simulink model "Safety_filter_obstacle_run"  (R2021b)
settings: Solver=ode4  StartTime=0.0  StopTime=30  FixedStep=0.01  RelTol=1e-3
settings Model: PacingRate=0.500000  Creator=14244039  LastModifiedBy=40335991
settings DebuggingCC: UnderSpecifiedDimensionMsg=warning

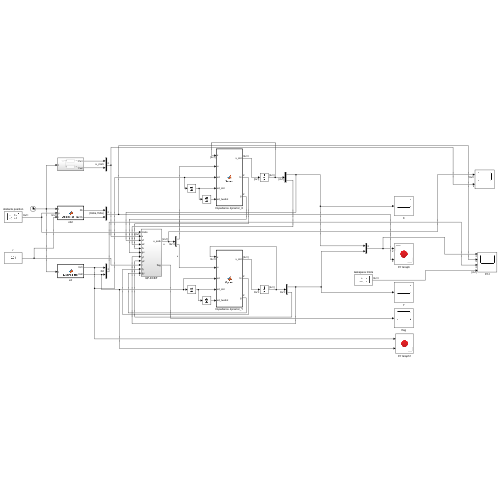
[thumbnail: Simulink's stored preview of the top-level diagram]
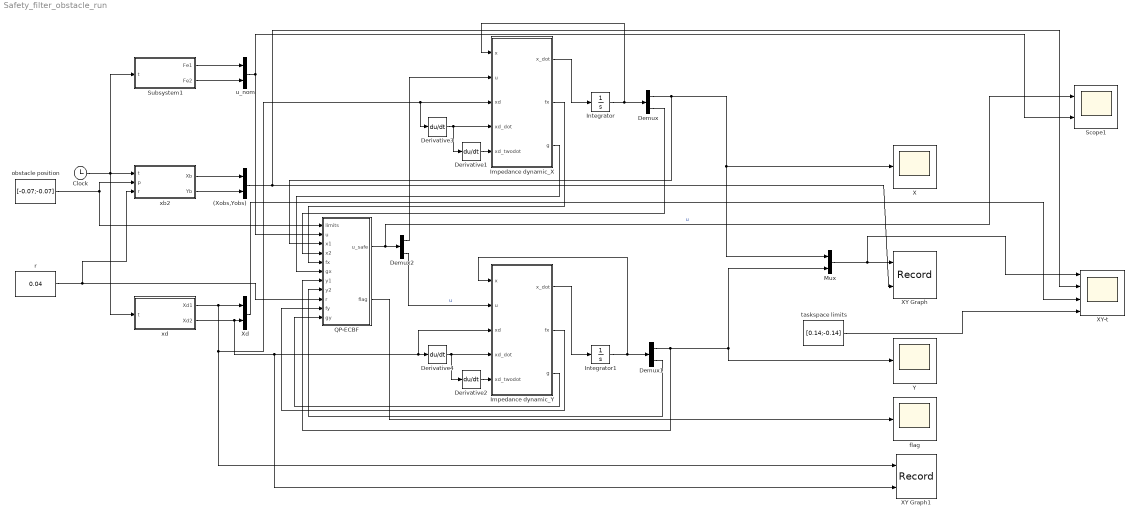
== system Safety_filter_obstacle_run ==
  (Xobs,Yobs) : Mux  Inputs=2
  Clock : Clock
  Demux : Demux  Outputs=2
  Demux1 : Demux  Outputs=2
  Demux2 : Demux  Outputs=2
  Derivative{1..4} (4 alike) : Derivative
  Impedance dynamic_X : MATLAB Function  TreatAsAtomicUnit=on
  Impedance dynamic_Y : MATLAB Function  TreatAsAtomicUnit=on
  Integrator : Integrator  InitialCondition=[0.14;0]
  Integrator1 : Integrator  InitialCondition=[0;0]
  Mux : Mux  Inputs=2
  QP-ECBF : Subsystem
  Scope1 : Scope  NumInputPorts=2
  Subsystem1 : Subsystem
  X : Scope
  XY Graph : Record  FileSettingsInternal="{\"entries\":[{\"content\":{\"excelSettings\":{\"content\":{},\"type\":\"Streamout.ExcelSettings\"}},\"type\":\"Streamout.FileSettingStorage\",\"uuid\":\"2cb9fd5d-0c84-4006-89a3-e297fa6ee1b5\"}],\"packageUris\":[\"http://schema.mathworks.com/mf0/streamout_blocks/R2020a\"],\"version\":\"1.0\"}"  Layout=[1 1]  SignalsInternal="{\"entries\":[{\"content\":{\"signals\":[{\"content\":{\"blockPath\":[\"Safety_filter_obstacle_run/XY Graph\"],\"channel\":[],\"dimensions\":[2],\"domain\":\"Safety_filter_obstacle_run/XY Graph\",\"hasChildren\":true,\"lineColor\":\"#fe330a\",\"plots\":[],\"port\":1,\"sid\":[\"\"],\"signalID\":5016,\"signalName\":\"Mux\"},\"type\":\"RecordBlkView.Signal\",\"uuid\":\"6b362bb2-f6dd-4a03-85b8-156c16026f8e\"},{\"content\":{\"blockPath\":[\"Safety_filter_obstacle_run/XY Graph\"],\"channel\":[1],\"dimensions\":[2],\"domain\":\"Safety_filter_obstacle_run/XY Graph\",\"lineColor\":\"#d95319\",\"parentID\":5016,\"plots\":[1],\"port\":1,\"sid\":[\"\"],\"signalID\":5017,\"signalName\":\"Mux\"},\"type\":\"RecordBlkView.Signal\",\"uuid\":\"500ae97e-7081-4371-a208-a6de7c56ece4\"},{\"content\":{\"blockPath\":[\"Safety_filter_obstacle_run/XY Graph\"],\"channel\":[],\"dimensions\":[2],\"domain\":\"Safety_filter_obstacle_run/XY Graph\",\"hasChildren\":true,\"lineColor\":\"#0072bd\",\"plots\":[],\"port\":2,\"sid\":[\"\"],\"signalID\":5021,\"signalName\":\"(Xobs,Yobs)\"},\"type\":\"RecordBlkView.Signal\",\"uuid\":\"f31b4382-cf55-47a1-8b18-86527234a350\"},{\"content\":{\"blockPath\":[\"Safety_filter_obstacle_run/XY Graph\"],\"channel\":[1],\"dimensions\":[2],\"domain\":\"Safety_filter_obstacle_run/XY Graph\",\"lineColor\":\"#7e2f8e\",\"parentID\":5021,\"plots\":[1],\"port\":2,\"sid\":[\"\"],\"signalID\":5022,\"signalName\":\"(Xobs,Yobs)\"},\"type\":\"RecordBlkView.Signal\",\"uuid\":\"742af8a8-3d57-45a7-b4dd-15d9969bab4c\"},{\"content\":{\"blockPath\":[\"Safety_filter_obstacle_run/XY Graph\"],\"channel\":[2],\"dimensions\":[2],\"domain\":\"Safety_filter_obstacle_run/XY Graph\",\"lineColor\":\"#a2142f\",\"parentID\":5016,\"plots\":[1],\"port\":1,\"sid\":[\"\"],\"signalID\":5035,\"signalName\":\"Mux\"},\"type\":\"RecordBlkView.Signal\",\"uuid\":\"5f11a2ec-fe27-4e67-93d5-fd7bb7e6a2c3\"},{\"content\":{\"blockPath\":[\"Safety_filter_obstacle_run/XY Graph\"],\"channel\":[2],\"dimensions\":[2],\"domain\":\"Safety_filter_obstacle_run/XY Graph\",\"lineColor\":\"#139fff\",\"parentID\":5021,\"plots\":[1],\"port\":2,\"sid\":[\"\"],\"signalID\":5036,\"signalName\":\"(Xobs,Yobs)\"},\"type\":\"RecordBlkView.Signal\",\"uuid\":\"66022486-a783-44e2-b1af-9294e060b914\"}]},\"type\":\"RecordBlkView.InputSignals\",\"uuid\":\"045e9bd8-92bd-4ba2-811b-fb3cc024f96b\"}],\"packageUris\":[\"http://schema.mathworks.com/mf0/streamout_blocks/R2020a\"],\"version\":\"1.0\"}"  VisualizationBindings="{\"xyplotplugin\":{\"info\":[{\"series\":[{\"bindingParametersList\":[{\"parameter\":\"X-Axis\",\"signalID\":5022,\"signalName\":\"(Xobs,Yobs)(1)\"},{\"parameter\":\"Y-Axis\",\"signalID\":5036,\"signalName\":\"(Xobs,Yobs)(2)\"}],\"seriesID\":588},{\"bindingParametersList\":[{\"parameter\":\"X-Axis\",\"signalID\":5017,\"signalName\":\"Mux(1)\"},{\"parameter\":\"Y-Axis\",\"signalID\":5035,\"signalName\":\"Mux(2)\"}],\"seriesID\":13609}],\"subplotID\":1}]}}"  CompatibilityTag=XY  st=-1
  XY Graph1 : Record  FileSettingsInternal="{\"entries\":[{\"content\":{\"excelSettings\":{\"content\":{},\"type\":\"Streamout.ExcelSettings\"}},\"type\":\"Streamout.FileSettingStorage\",\"uuid\":\"2cef4229-92dc-4655-bad0-2b3161d59ac8\"}],\"packageUris\":[\"http://schema.mathworks.com/mf0/streamout_blocks/R2020a\"],\"version\":\"1.0\"}"  Layout=[1 1]  SignalsInternal="{\"entries\":[{\"content\":{\"signals\":[{\"content\":{\"blockPath\":[\"Safety_filter_obstacle_run/XY Graph1\"],\"channel\":[],\"dimensions\":[1],\"domain\":\"Safety_filter_obstacle_run/XY Graph1\",\"lineColor\":\"#a2142f\",\"plots\":[1],\"port\":1,\"sid\":[\"\"],\"signalID\":5026,\"signalName\":\"xd:1\"},\"type\":\"RecordBlkView.Signal\",\"uuid\":\"d43ebe69-de7a-456f-bba9-24daebe6bc4b\"},{\"content\":{\"blockPath\":[\"Safety_filter_obstacle_run/XY Graph1\"],\"channel\":[],\"dimensions\":[1],\"domain\":\"Safety_filter_obstacle_run/XY Graph1\",\"lineColor\":\"#139fff\",\"plots\":[1],\"port\":2,\"sid\":[\"\"],\"signalID\":5030,\"signalName\":\"xd:2\"},\"type\":\"RecordBlkView.Signal\",\"uuid\":\"3ab767b2-3981-4008-8a03-ee9b94162d99\"}]},\"type\":\"RecordBlkView.InputSignals\",\"uuid\":\"ec3b1ac5-575a-40f9-bce4-3baa89b708d6\"}],\"packageUris\":[\"http://schema.mathworks.com/mf0/streamout_blocks/R2020a\"],\"version\":\"1.0\"}"  VisualizationBindings="{\"xyplotplugin\":{\"info\":[{\"series\":[{\"bindingParametersList\":[{\"parameter\":\"X-Axis\",\"signalID\":5026,\"signalName\":\"xd:1\"},{\"parameter\":\"Y-Axis\",\"signalID\":5030,\"signalName\":\"xd:2\"}],\"seriesID\":51409}],\"subplotID\":1}]}}"  CompatibilityTag=XY
  XY-t : Scope  NumInputPorts=4
  Xd : Mux  Inputs=2
  Y : Scope
  flag : Scope
  obstacle position : Constant  Value=[-0.07;-0.07]  VectorParams1D=off  SampleTime=-1
  r : Constant  Value=0.04  VectorParams1D=off  SampleTime=-1
  taskspace limits : Constant  Value=[0.14;-0.14]  VectorParams1D=off  SampleTime=-1
  u_nom : Mux  Inputs=2
  xb2 : MATLAB Function  TreatAsAtomicUnit=on
  xd : MATLAB Function  TreatAsAtomicUnit=on
  wires:
  Subsystem1/1(Fe1) -> u_nom/1
  Clock/1 -> xd/1(t), xb2/1(t), Subsystem1/1(t)
  Derivative3/1 -> Impedance dynamic_X/4(xd_dot), Derivative1/1
  Derivative1/1 -> Impedance dynamic_X/5(xd_twodot)
  Impedance dynamic_X/1(x_dot) -> Integrator/1
  Integrator/1 -> Demux/1, Impedance dynamic_X/1(x)
  Demux/1 -> QP-ECBF/3(x1), Mux/1, X/1
  Demux2/2 -> Impedance dynamic_Y/2(u)  "u"
  Demux1/1 -> QP-ECBF/7(y1), Y/1, Mux/2
  xd/2(Xd2) -> XY Graph1/2, Impedance dynamic_Y/3(xd), Derivative4/1, Xd/2
  Impedance dynamic_Y/1(x_dot) -> Integrator1/1
  Derivative4/1 -> Impedance dynamic_Y/4(xd_dot), Derivative2/1
  Derivative2/1 -> Impedance dynamic_Y/5(xd_twodot)
  Integrator1/1 -> Demux1/1, Impedance dynamic_Y/1(x)
  Subsystem1/2(Fe2) -> u_nom/2
  xb2/1(Xb) -> (Xobs,Yobs)/1
  xb2/2(Yb) -> (Xobs,Yobs)/2
  Mux/1 -> XY-t/1, XY Graph/1
  (Xobs,Yobs)/1 -> XY-t/2, XY Graph/2
  QP-ECBF/1(u_safe) -> Scope1/1, Demux2/1  "u"
  Demux2/1 -> Impedance dynamic_X/2(u)
  obstacle position/1 -> xb2/2(p), QP-ECBF/1(limits)
  u_nom/1 -> QP-ECBF/2(u), Scope1/2
  Demux/2 -> QP-ECBF/4(x2)
  Impedance dynamic_X/2(fx) -> QP-ECBF/5(fx)
  Impedance dynamic_X/3(g) -> QP-ECBF/6(gx)
  Demux1/2 -> QP-ECBF/8(y2)
  r/1 -> xb2/3(r), QP-ECBF/9(r)
  QP-ECBF/2(flag) -> flag/1
  Impedance dynamic_Y/2(fx) -> QP-ECBF/10(fy)
  Impedance dynamic_Y/3(g) -> QP-ECBF/11(gy)
  xd/1(Xd1) -> XY Graph1/1, Impedance dynamic_X/3(xd), Derivative3/1, Xd/1
  Xd/1 -> XY-t/3
  taskspace limits/1 -> XY-t/4

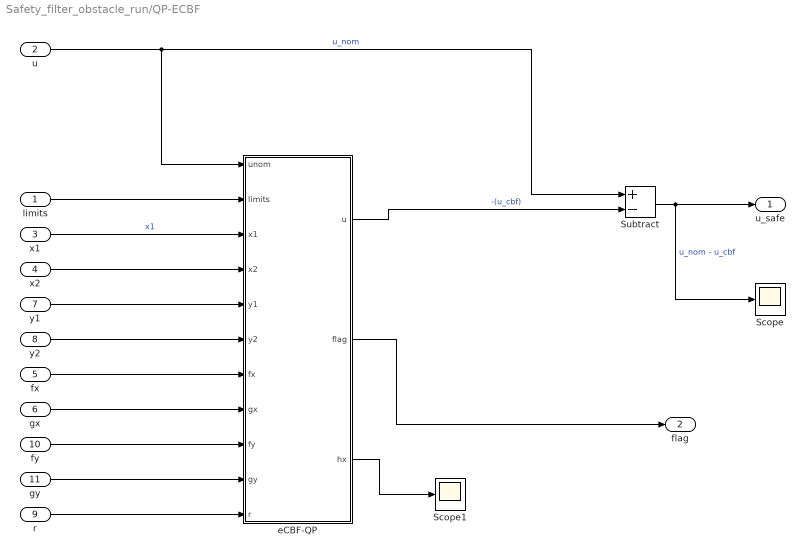
== system Safety_filter_obstacle_run/QP-ECBF ==
  limits : Inport
  u : Inport  Port=2
  x1 : Inport  Port=3
  x2 : Inport  Port=4
  fx : Inport  Port=5
  gx : Inport  Port=6
  y1 : Inport  Port=7
  y2 : Inport  Port=8
  r : Inport  Port=9
  fy : Inport  Port=10
  gy : Inport  Port=11
  Scope : Scope
  Scope1 : Scope
  Subtract : Sum  Inputs=+-
  eCBF-QP : MATLAB Function  TreatAsAtomicUnit=on
  u_safe : Outport
  flag : Outport  Port=2
  wires:
  x2/1 -> eCBF-QP/4(x2)
  limits/1 -> eCBF-QP/2(limits)
  u/1 -> eCBF-QP/1(unom), Subtract/1  "u_nom"
  x1/1 -> eCBF-QP/3(x1)  "x1"
  eCBF-QP/1(u) -> Subtract/2  "-(u_cbf)"
  Subtract/1 -> u_safe/1, Scope/1  "u_nom - u_cbf"
  fx/1 -> eCBF-QP/7(fx)
  gx/1 -> eCBF-QP/8(gx)
  eCBF-QP/2(flag) -> flag/1
  y1/1 -> eCBF-QP/5(y1)
  y2/1 -> eCBF-QP/6(y2)
  r/1 -> eCBF-QP/11(r)
  eCBF-QP/3(hx) -> Scope1/1
  fy/1 -> eCBF-QP/9(fy)
  gy/1 -> eCBF-QP/10(gy)

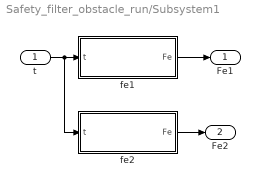
== system Safety_filter_obstacle_run/Subsystem1 ==
  t : Inport
  fe1 : MATLAB Function  TreatAsAtomicUnit=on
  fe2 : MATLAB Function  TreatAsAtomicUnit=on
  Fe1 : Outport
  Fe2 : Outport  Port=2
  wires:
  fe1/1(Fe) -> Fe1/1
  fe2/1(Fe) -> Fe2/1
  t/1 -> fe2/1(t), fe1/1(t)

== matlab function Safety_filter_obstacle_run/Impedance dynamic_Y ==
  data: x input size=[2 1]; u input; x_dot output size=[2 1]; xd input; xd_dot input; xd_twodot input; fx output; g output
function [x_dot,fx,g] = System(x,u,xd,xd_dot,xd_twodot)

    km = 20;
    kb = 20;                                                       
    kk = 100;
    fx = [x(2);
        -(1/km)*(kb*(x(2)-xd_dot)+kk*(x(1)-xd)-km*xd_twodot)];
    g = [0;km^(-1)];
    x_dot = fx + g*u;
end

== matlab function Safety_filter_obstacle_run/Subsystem1/fe1 ==
  data: t input; Fe output
function Fe  = External_force(t)

   Fe = 0*(t<4|t>=11) + (1-cos(pi*t))*(t>=4&t<5) + 2*(t>=5&t<10) + (1+cos(pi*t))*(t>=10&t<11);

end

== matlab function Safety_filter_obstacle_run/Subsystem1/fe2 ==
  data: t input; Fe output
function Fe  = External_force(t)

   Fe = 0*(t<4|t>=11) + 2*(1-cos(pi*t))*(t>=4&t<5) + 4*(t>=5&t<10) + 2*(1+cos(pi*t))*(t>=10&t<11);

end

== matlab function Safety_filter_obstacle_run/xd ==
  data: t input; Xd1 output; Xd2 output
function [Xd1, Xd2] = Desired_traj(t)

    Xd1=0.14*cos(0.5*t);
    Xd2=0.14*sin(0.5*t);
    
end

== matlab function Safety_filter_obstacle_run/QP-ECBF/eCBF-QP ==
  settings: updateMethod=DISCRETE
  data: unom input; limits input; u output size=[2 1]; x1 input; x2 input; y1 input; y2 input; fx input; gx input; fy input; gy input; flag output; r input; hx output
function [u,flag,hx] = fcn(unom, limits, x1, x2,y1 ,y2 ,fx,gx,fy,gy,r)
    %% Obstacle position
    X_obs    = limits(1);
    Y_obs    = limits(2);
    fe_x = unom(1);
    fe_y = unom(2);
    %% ECBF Gains
    k1 = 70;
    k2 = 700;
    r = r+0.01;
    %% CBF 
    hx      = (x1 - X_obs)^2 + (y1 - Y_obs)^2 - r^2 ; 
    Lfhx    = 2*(x1 - X_obs)*x2 + 2*(y1 - Y_obs)*y2;
    L2fhx_unom = 2*(x1 - X_obs)*( gx(2)*fe_x) + 2*(y1 - Y_obs)*( gy(2)*fe_y) ;

    L2fhx_usafe_x = 2*(x1 - X_obs)*gx(2);
    L2fhx_usafe_y = 2*(y1 - Y_obs)*gy(2);
   

    H       = [2 0; 0 2];
    f       = [0;0]; 
    
    A       = [L2fhx_usafe_x, L2fhx_usafe_y]; 
            
    b       = [L2fhx_unom + k1*Lfhx + k2*hx];
    X   = [0;0];
    flag = 0;
    coder.extrinsic('quadprog');
    [output, ~, flag]   = quadprog(H,f,A,b,[],[],[],[]);

    if flag == 1
        X = output;
    else
        X   = [0;0];
    end
    
%Function outputs
    u = X; 
end

== matlab function Safety_filter_obstacle_run/Impedance dynamic_X ==
  data: x input size=[2 1]; u input; x_dot output size=[2 1]; xd input; xd_dot input; xd_twodot input; fx output; g output
function [x_dot,fx,g] = System(x,u,xd,xd_dot,xd_twodot)

    km = 20;
    kb = 20;                                                       
    kk = 100;
    fx = [x(2);
        -(1/km)*(kb*(x(2)-xd_dot)+kk*(x(1)-xd)-km*xd_twodot)];
    g = [0;km^(-1)];
    x_dot = fx + g*u;
end

== matlab function Safety_filter_obstacle_run/xb2 ==
  data: t input; Xb output; Yb output; p input; r input
function [Xb,Yb]  = Obstacles_traj(t,p,r)

Xb =  p(1) + r*cos(t);
Yb =  p(2) + r*sin(t);
    
end
